simulink model "ModeRspCaller"  (R2018b)
settings: Solver=FixedStepDiscrete  StartTime=0.0  StopTime=10.0  RelTol=1e-3
undefined symbols (not defined in the file or in its folder): CHM2Ctrl_Cal, MdXX_RspOutCommCalc_Cal, MdXX_RspToNetWork_Cal, MdXX_Status_Cal, MdXX_StatusToNetWork_Cal, SRSModeState_Cal, SRSSwIndCtrl_Cal, StPassCmprtMdHMIDisCmdCalc_Cal
settings Model: Creator=sn2xws  LastModifiedBy=sn2xws
settings DataIOCC: SaveFormat=StructureWithTime
settings OptimizationCC: DefaultParameterBehavior=Inlined  EnhancedBackFolding=on  PassReuseOutputArgsAs=Individual arguments  ZeroExternalMemoryAtStartup=off  ZeroInternalMemoryAtStartup=off  OptimizeBlockOrder=speed  DifferentSizesBufferReuse=on  OptimizationCustomize=off
settings DebuggingCC: ParameterTunabilityLossMsg=error
settings SFSimCC: MATLABDynamicMemAlloc=off
settings RTWCC: SystemTargetFile=autosar.tlc  GenCodeOnly=on  TemplateMakefile=ert_default_tmf  Description=AUTOSAR  GenerateReport=on  IncludeHyperlinkInReport=on  LaunchReport=on  GenerateTraceInfo=on  GenerateTraceReport=on  GenerateTraceReportSl=on  GenerateTraceReportSf=on  GenerateTraceReportEml=on  GenerateCodeMetricsReport=on
settings CodeAppCC: ForceParamTrailComments=on  IgnoreCustomStorageClasses=off  OperatorAnnotations=on  SimulinkDataObjDesc=on  SFDataObjDesc=on  InsertBlockDesc=on
settings STFCustomTargetCC: TargetLangStandard=C99 (ISO)  MultiwordLength=256  ParMdlRefBuildCompliant=on  CompOptLevelCompliant=on  IncludeMdlTerminateFcn=off  CombineOutputUpdateFcns=on  SuppressErrorStatus=on  ERTCustomFileBanners=on  SupportNonFinite=off  SupportComplex=off  SupportContinuousTime=off  SupportNonInlinedSFcns=off  RemoveResetFunc=on  MATLABClassNameForMDSCustomization=Simulink.SoftwareTarget.ERTCustomization  AutosarCompliant=on  UseToolchainInfoCompliant=on  LookupTableObjectStructAxisOrder=2,1,3,4,...  LUTObjectStructOrderEvenSpacing=Size,Table,Breakpoints  SystemTargetFile=autosar.tlc
settings ERTTargetCC: TargetLangStandard=C99 (ISO)  ConcurrentExecutionCompliant=off  IncludeMdlTerminateFcn=off  SuppressErrorStatus=on  SupportNonFinite=off  SupportComplex=off  ModelStepFunctionPrototypeControlCompliant=off  CPPClassGenCompliant=off  AutosarCompliant=on  LookupTableObjectStructAxisOrder=2,1,3,4,...  LUTObjectStructOrderEvenSpacing=Size,Table,Breakpoints  InlinedParameterPlacement=NonHierarchical  ERTCustomFileTemplate=example_file_process.tlc  ERTFilePackagingFormat=Compact

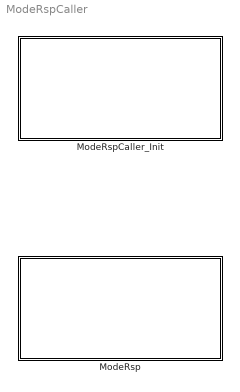
== system ModeRspCaller ==
  ModeRsp : Subsystem
  ModeRspCaller_Init : Subsystem

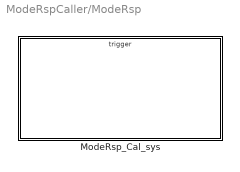
== system ModeRspCaller/ModeRsp ==
  ModeRsp_Cal_sys : Subsystem

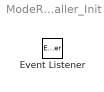
== system ModeRspCaller/ModeRspCaller_Init ==
  Event Listener : EventListener  EventName=reset

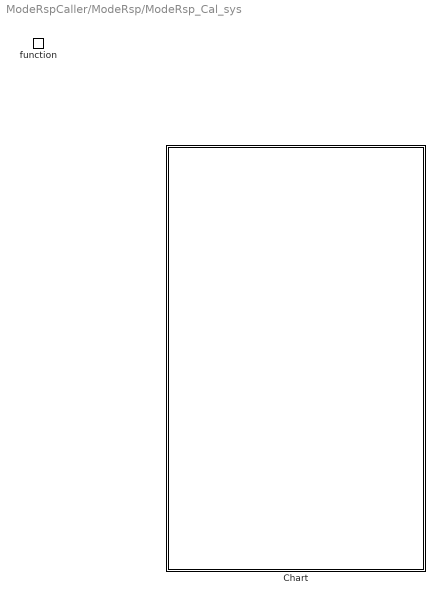
== system ModeRspCaller/ModeRsp/ModeRsp_Cal_sys ==
  function : TriggerPort  TriggerType=function-call  IsSimulinkFunction=on  FunctionName=ModeRsp_Cal  VariantControl=(inherit)
  Chart : Stateflow chart  TreatAsAtomicUnit=on

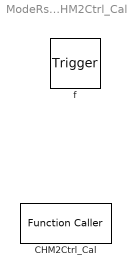
== system ModeRspCaller/ModeRsp/ModeRsp_Cal_sys/Chart/CHM2Ctrl_Cal ==
  f : TriggerPort  TriggerType=function-call  VariantControl=(inherit)
      settings: CopyFcn=Stateflow.SLINSF.SimulinkMan.removeBlockPreDeleteFcn  PreDeleteFcn=Stateflow.SLINSF.SimulinkMan.unsafePredeleteFcn
  CHM2Ctrl_Cal : FunctionCaller  FunctionPrototype=CHM2Ctrl_Cal()

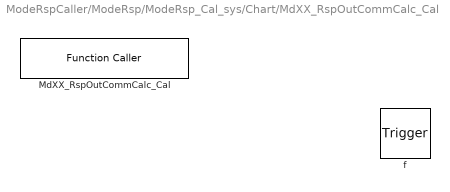
== system ModeRspCaller/ModeRsp/ModeRsp_Cal_sys/Chart/MdXX_RspOutCommCalc_Cal ==
  f : TriggerPort  TriggerType=function-call  VariantControl=(inherit)
      settings: CopyFcn=Stateflow.SLINSF.SimulinkMan.removeBlockPreDeleteFcn  PreDeleteFcn=Stateflow.SLINSF.SimulinkMan.unsafePredeleteFcn
  MdXX_RspOutCommCalc_Cal : FunctionCaller  FunctionPrototype=MdXX_RspOutCommCalc_Cal()

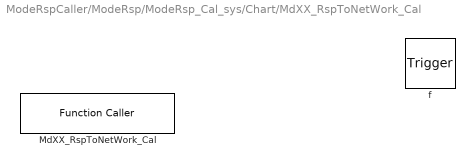
== system ModeRspCaller/ModeRsp/ModeRsp_Cal_sys/Chart/MdXX_RspToNetWork_Cal ==
  f : TriggerPort  TriggerType=function-call  VariantControl=(inherit)
      settings: CopyFcn=Stateflow.SLINSF.SimulinkMan.removeBlockPreDeleteFcn  PreDeleteFcn=Stateflow.SLINSF.SimulinkMan.unsafePredeleteFcn
  MdXX_RspToNetWork_Cal : FunctionCaller  FunctionPrototype=MdXX_RspToNetWork_Cal()

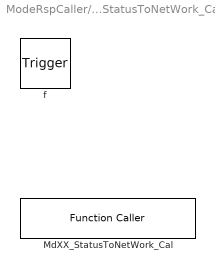
== system ModeRspCaller/ModeRsp/ModeRsp_Cal_sys/Chart/MdXX_StatusToNetWork_Cal ==
  f : TriggerPort  TriggerType=function-call  VariantControl=(inherit)
      settings: CopyFcn=Stateflow.SLINSF.SimulinkMan.removeBlockPreDeleteFcn  PreDeleteFcn=Stateflow.SLINSF.SimulinkMan.unsafePredeleteFcn
  MdXX_StatusToNetWork_Cal : FunctionCaller  FunctionPrototype=MdXX_StatusToNetWork_Cal()

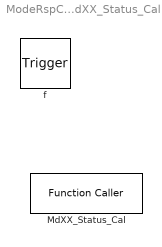
== system ModeRspCaller/ModeRsp/ModeRsp_Cal_sys/Chart/MdXX_Status_Cal ==
  f : TriggerPort  TriggerType=function-call  VariantControl=(inherit)
      settings: CopyFcn=Stateflow.SLINSF.SimulinkMan.removeBlockPreDeleteFcn  PreDeleteFcn=Stateflow.SLINSF.SimulinkMan.unsafePredeleteFcn
  MdXX_Status_Cal : FunctionCaller  FunctionPrototype=MdXX_Status_Cal()

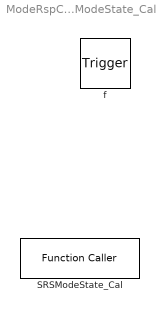
== system ModeRspCaller/ModeRsp/ModeRsp_Cal_sys/Chart/SRSModeState_Cal ==
  f : TriggerPort  TriggerType=function-call  VariantControl=(inherit)
      settings: CopyFcn=Stateflow.SLINSF.SimulinkMan.removeBlockPreDeleteFcn  PreDeleteFcn=Stateflow.SLINSF.SimulinkMan.unsafePredeleteFcn
  SRSModeState_Cal : FunctionCaller  FunctionPrototype=SRSModeState_Cal()

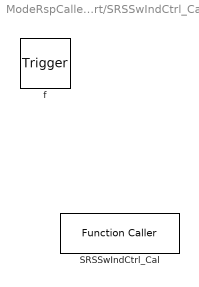
== system ModeRspCaller/ModeRsp/ModeRsp_Cal_sys/Chart/SRSSwIndCtrl_Cal ==
  f : TriggerPort  TriggerType=function-call  VariantControl=(inherit)
      settings: CopyFcn=Stateflow.SLINSF.SimulinkMan.removeBlockPreDeleteFcn  PreDeleteFcn=Stateflow.SLINSF.SimulinkMan.unsafePredeleteFcn
  SRSSwIndCtrl_Cal : FunctionCaller  FunctionPrototype=SRSSwIndCtrl_Cal()

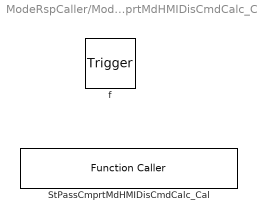
== system ModeRspCaller/ModeRsp/ModeRsp_Cal_sys/Chart/StPassCmprtMdHMIDisCmdCalc_Cal ==
  f : TriggerPort  TriggerType=function-call  VariantControl=(inherit)
      settings: CopyFcn=Stateflow.SLINSF.SimulinkMan.removeBlockPreDeleteFcn  PreDeleteFcn=Stateflow.SLINSF.SimulinkMan.unsafePredeleteFcn
  StPassCmprtMdHMIDisCmdCalc_Cal : FunctionCaller  FunctionPrototype=StPassCmprtMdHMIDisCmdCalc_Cal()

== stateflow chart ModeRspCaller/ModeRsp/ModeRsp_Cal_sys/Chart ==
  state MdXX_RspOutCommCalc_Cal [function]
  state MdXX_Status_Cal [function]
  state SRSModeState_Cal [function]
  state CHM2Ctrl_Cal [function]
  state StPassCmprtMdHMIDisCmdCalc_Cal [function]
  state MdXX_RspToNetWork_Cal [function]
  state MdXX_StatusToNetWork_Cal [function]
  state SRSSwIndCtrl_Cal [function]
  (default) -> (junction 3)
  (junction 3) -> (junction 5) : {
      | MdXX_RspOutCommCalc_Cal();
      | MdXX_Status_Cal();
      | SRSModeState_Cal();
      | CHM2Ctrl_Cal();
      | StPassCmprtMdHMIDisCmdCalc_Cal();
      | MdXX_RspToNetWork_Cal();
      | MdXX_StatusToNetWork_Cal();
      | SRSSwIndCtrl_Cal();
      | }
